simulink model "gesamtkonzept1"  (R2016b)
settings: Solver=VariableStepAuto  StartTime=0.0  StopTime=10.0  RelTol=1e-3
settings Model: Creator=Fritz  LastModifiedBy=Fritz

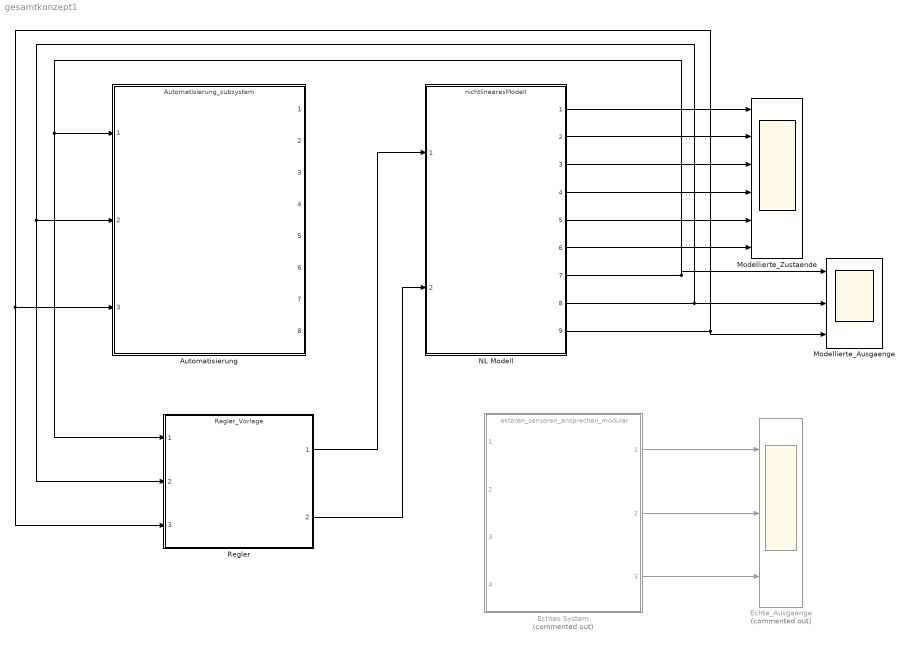
== system gesamtkonzept1 ==
  Automatisierung : ModelReference  ModelNameDialog=Automatisierung_subsystem.slx  SimulationMode=Normal  ModelReferenceVersion=1.27
  Echte_Ausgaenge : Scope  Commented=on  NumInputPorts=3
  Echtes System : ModelReference  Commented=on  ModelNameDialog=aktoren_sensoren_ansprechen_modular.slx  SimulationMode=Normal  ModelReferenceVersion=1.21
  Modellierte_Ausgaenge : Scope  NumInputPorts=3
  Modellierte_Zustaende : Scope  NumInputPorts=6
  NL Modell : ModelReference  ModelNameDialog=nichtlinearesModell.slx  SimulationMode=Normal  ModelReferenceVersion=1.3
  Regler : ModelReference  ModelNameDialog=Regler_Vorlage.slx  SimulationMode=Normal  ModelReferenceVersion=1.1
  wires:
  NL Modell/1 -> Modellierte_Zustaende/1
  NL Modell/2 -> Modellierte_Zustaende/2
  NL Modell/3 -> Modellierte_Zustaende/3
  NL Modell/4 -> Modellierte_Zustaende/4
  NL Modell/5 -> Modellierte_Zustaende/5
  NL Modell/6 -> Modellierte_Zustaende/6
  NL Modell/7 -> Automatisierung/1, Regler/1, Modellierte_Ausgaenge/1
  NL Modell/8 -> Automatisierung/2, Regler/2, Modellierte_Ausgaenge/2
  NL Modell/9 -> Automatisierung/3, Regler/3, Modellierte_Ausgaenge/3
  Regler/1 -> NL Modell/1
  Regler/2 -> NL Modell/2
  Echtes System/1 -> Echte_Ausgaenge/1
  Echtes System/2 -> Echte_Ausgaenge/2
  Echtes System/3 -> Echte_Ausgaenge/3
